simulink model "Test_PMSM_PI_fixed_MTPA"  (R2024b)
settings: Solver=ode45  StartTime=0.0  StopTime=10e-3  FixedStep=Ts  MaxStep=TCs/2  RelTol=1e-3
values from neighbouring files (symbols this model uses):
  Ki_Id = 5.274e3    (= 5274)    [init_params.m]
  Ki_Iq = 9.846e3    (= 9846)    [init_params.m]
  Kp_Id = 4.746    [init_params.m]
  Kp_Iq = 8.861    [init_params.m]
  p = 4    [init_params.m]
  TCs = 1/Fs    (= 0.0001)    [init_params.m]
  Tref = 60    [init_params.m]
undefined symbols (not defined in the file or in its folder): Mot, plecs
libraries: eeTransforms x3, slpidlib x2, simulink x1, spsabctoAlphaBetaZeroLib x1
settings Model: Creator=juan  LastModifiedBy=jd
settings RTWCC: GPUComputeCapability=3.5

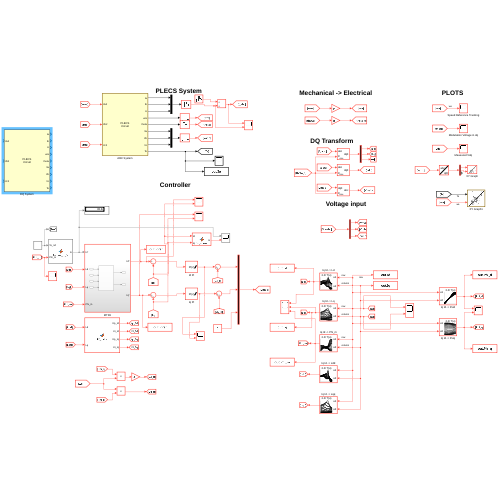
[thumbnail: Simulink's stored preview of the top-level diagram]
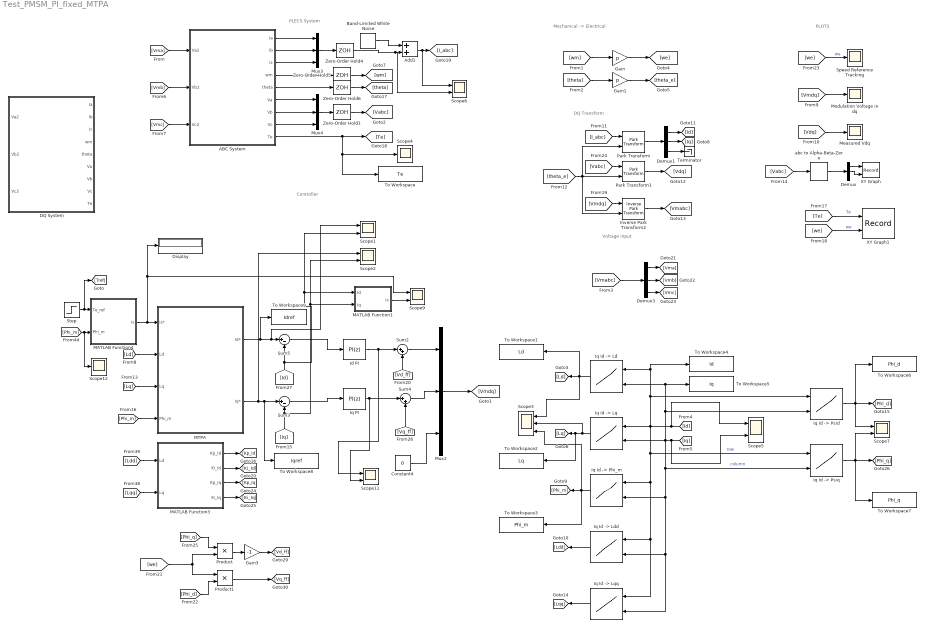
== system Test_PMSM_PI_fixed_MTPA ==
  note: Controller
  note: PLECS System
  note: Mechanical -> Electrical
  note: DQ Transform
  note: PLOTS
  note: Voltage input
  ABC System : Subsystem  LoadFcn=plecs('sl', 200);  InitFcn=plecs('sl', 214);  StartFcn=plecs('sl', 208);  StopFcn=plecs('sl', 209);  mask(PlecsCircuit){PLECSData=<binary blob, 53316 chars, not shown>}
      mask prompts: PLECSData "PLECS Data (Do not delete or modify!)"
      mask init:
      | % PLACE CUSTOM INITIALIZATIONS ABOVE
      | % DO NOT REMOVE
      | plecs('sl', 215);
      | % DO NOT REMOVE
      settings: CopyFcn=plecs('sl', 203);  DeleteFcn=plecs('sl', 205);  UndoDeleteFcn=plecs('sl', 206);  PreSaveFcn=plecs('sl', 211);  PostSaveFcn=plecs('sl', 201);  NameChangeFcn=plecs('sl', 210);  DestroyFcn=plecs('sl', 207);  PreCopyFcn=plecs('sl', 216);  OpenFcn=plecs('sl', 202);  ErrorFcn=plerrorfcn
      mask Help: eval('plecs(''help'', ''qthelp:///creatingacircuit.html'')')
      mask Display: disp('PLECS\nCircuit')
  Add1 : Sum
  Band-Limited White Noise : simulink/Sources/Band-Limited White Noise  Cov=[1]  Ts=TCs  seed=[23341]
  Constant4 : Constant  Value=0  SampleTime=TCs
  DQ System : Subsystem  LoadFcn=plecs('sl', 200);  InitFcn=plecs('sl', 214);  StartFcn=plecs('sl', 208);  StopFcn=plecs('sl', 209);  mask(PlecsCircuit){PLECSData=<binary blob, 50632 chars, not shown>}
      mask prompts: PLECSData "PLECS Data (Do not delete or modify!)"
      mask init:
      | % PLACE CUSTOM INITIALIZATIONS ABOVE
      | % DO NOT REMOVE
      | plecs('sl', 215);
      | % DO NOT REMOVE
      settings: CopyFcn=plecs('sl', 203);  DeleteFcn=plecs('sl', 205);  UndoDeleteFcn=plecs('sl', 206);  PreSaveFcn=plecs('sl', 211);  PostSaveFcn=plecs('sl', 201);  NameChangeFcn=plecs('sl', 210);  DestroyFcn=plecs('sl', 207);  PreCopyFcn=plecs('sl', 216);  OpenFcn=plecs('sl', 202);  ErrorFcn=plerrorfcn
      mask Help: eval('plecs(''help'', ''qthelp:///creatingacircuit.html'')')
      mask Display: disp('PLECS\nCircuit')
  Demux : Demux  Outputs=3
  Demux1 : Demux  Outputs=3
  Demux3 : Demux  Outputs=3
  Display : Display
  Gain : Gain  Gain=p
  Gain1 : Gain  Gain=p
  Gain3 : Gain  Gain=-1
  Id PI : slpidlib/PID Controller  Controller=PI  Form=Parallel  TimeDomain=Discrete-time  UseExternalTs=off  SampleTime=TCs  IntegratorMethod=Forward Euler  FilterMethod=Forward Euler  ControllerParametersSource=internal  P=Kp_Id  I=Ki_Id  UseKiTs=off  D=0  UseExternalDerivativeSource=off  N=100  UseFilter=on  TunerSelectOption=Transfer Function Based (PID Tuner App)  InitialConditionSource=internal  InitialConditionForIntegrator=0  InitialConditionForFilter=0  DifferentiatorICPrevScaledInput=0  ExternalReset=none  TrackingMode=off  Kt=1  LimitOutput=on  SatLimitsSource=internal  UpperSaturationLimit=310/sqrt(3)  LowerSaturationLimit=-310/sqrt(3)  LinearizeAsGain=on  AntiWindupMode=clamping  Kb=1  LimitIntegrator=off  UpperIntegratorSaturationLimit=inf  LowerIntegratorSaturationLimit=-inf  POutMin=[]  POutMax=[]  IOutMin=[]  IOutMax=[]  DOutMin=[]  DOutMax=[]  NOutMin=[]  NOutMax=[]  SumOutMin=[]  SumOutMax=[]  SaturationOutMin=[]  SaturationOutMax=[]  PParamMin=[]  PParamMax=[]  IParamMin=[]  IParamMax=[]  DParamMin=[]  DParamMax=[]  NParamMin=[]  NParamMax=[]  KbParamMin=[]  KbParamMax=[]  KtParamMin=[]  KtParamMax=[]  KbOutMin=[]  KbOutMax=[]  KtOutMin=[]  KtOutMax=[]  IntegratorOutMin=[]  IntegratorOutMax=[]  FilterOutMin=[]  FilterOutMax=[]  SumI1OutMin=[]  SumI1OutMax=[]  SumI2OutMin=[]  SumI2OutMax=[]  SumI3OutMin=[]  SumI3OutMax=[]  SumI4OutMin=[]  SumI4OutMax=[]  SumDOutMin=[]  SumDOutMax=[]  DifferentiatorOutMin=[]  DifferentiatorOutMax=[]  FilterDiffOutCoefMin=[]  FilterDiffOutCoefMax=[]  ReciprocalOutMin=[]  ReciprocalOutMax=[]  SumDenOutMin=[]  SumDenOutMax=[]  SumNumOutMin=[]  SumNumOutMax=[]  DivideOutMin=[]  DivideOutMax=[]  UdiffTsProdOutMin=[]  UdiffTsProdOutMax=[]  NTsProdOutMin=[]  NTsProdOutMax=[]  UintegralTsProdOutMin=[]  UintegralTsProdOutMax=[]  UngainTsProdOutMin=[]  UngainTsProdOutMax=[]  ClampingZeroOutDataTypeStr=Inherit: Inherit via back propagation  ClampingZeroOutMin=[]  ClampingZeroOutMax=[]  FilterDenConstantOutDataTypeStr=Inherit: Inherit via back propagation  FilterDenConstantOutMin=[]  FilterDenConstantOutMax=[]  PCopyOutDataTypeStr=Inherit: Inherit via back propagation  PCopyOutMin=[]  PCopyOutMax=[]  NCopyOutDataTypeStr=Inherit: Inherit via back propagation  NCopyOutMin=[]  NCopyOutMax=[]  IntegratorContinuousStateAttributes=''  IntegratorStateMustResolveToSignalObject=off  IntegratorRTWStateStorageClass=Auto  FilterContinuousStateAttributes=''  FilterStateMustResolveToSignalObject=off  FilterRTWStateStorageClass=Auto  ParallelPVariant=InternalParameters  IdealPVariant=Disabled  IVariant=InternalParameters  DVariant=Disabled  IntegratorVariant=Discrete  SatVariant=Enabled  AWVariant=DiscClampingParallel  PCopyVariant=Disabled  TRVariant=Disabled  FdbkBlocksVariant=Forward  IdealPFdbkVariant=Disabled  SatFdbkVariant=Disabled  DerivativeFilterVariant=Disabled  NVariant=Disabled  NCopyVariant=Disabled_SignalSpec  FilterICVariant=Disabled  IntegratorICVariant=InternalICs  ExternalResetVariant=Disabled  TRSumVariant=Passthrough  SumFdbkVariant=Disabled  SumVariant=Sum_PI  TsampFilterVariant=InternalTs  TsampNgainVariant=Passthrough  TsampIntegralVariant=Disabled_SignalSpec  ExternalSaturationOutDataTypeStr=Inherit: Same as second input  DerivativeSourceVariant=Disabled  PreIntVariant=InternalPreInt
  Inverse Park Transform2 : eeTransforms/Inverse Park Transform  AxisAlignment=D-axis  PowerInvariant=off
      settings: LibrarySourceBlock=|
      | ee_sl_lib/Mathematical
      | Transforms/Inverse
      | Park Transform
  "Iq Id -> Ld" : Lookup_n-D  BreakpointsForDimension1=Mot.mag_t.imd  BreakpointsForDimension2=Mot.mag_t.imq  Table=Mot.mag_t.Lmidd+Mot.mag_t.Lmidq  InternalRulePriority=Speed  RndMeth=Simplest
      settings: InputPortMap=u0,u1
  "Iq Id -> Ldd" : Lookup_n-D  BreakpointsForDimension1=Mot.mag_t.imd  BreakpointsForDimension2=Mot.mag_t.imq  Table=Mot.mag_t.Lmidd  InternalRulePriority=Speed  RndMeth=Simplest
      settings: InputPortMap=u0,u1
  "Iq Id -> Lq" : Lookup_n-D  BreakpointsForDimension1=Mot.mag_t.imd  BreakpointsForDimension2=Mot.mag_t.imq  Table=Mot.mag_t.Lmiqq+Mot.mag_t.Lmidq  InternalRulePriority=Speed  RndMeth=Simplest
      settings: InputPortMap=u0,u1
  "Iq Id -> Lqq" : Lookup_n-D  BreakpointsForDimension1=Mot.mag_t.imd  BreakpointsForDimension2=Mot.mag_t.imq  Table=Mot.mag_t.Lmiqq  InternalRulePriority=Speed  RndMeth=Simplest
      settings: InputPortMap=u0,u1
  "Iq Id -> Phi_m" : Lookup_n-D  BreakpointsForDimension1=Mot.mag_t.imd  BreakpointsForDimension2=Mot.mag_t.imq  Table=Mot.mag_t.Psid - (Mot.mag_t.Lmidd + Mot.mag_t.Lmidq).*Mot.mag_t.imd'  InternalRulePriority=Speed  RndMeth=Simplest
      settings: InputPortMap=u0,u1
  "Iq Id -> Psid" : Lookup_n-D  BreakpointsForDimension1=Mot.mag_t.imd  BreakpointsForDimension2=Mot.mag_t.imq  Table=Mot.mag_t.Psid  InternalRulePriority=Speed  RndMeth=Simplest
      settings: InputPortMap=u0,u1
  "Iq Id -> Psiq" : Lookup_n-D  BreakpointsForDimension1=Mot.mag_t.imd  BreakpointsForDimension2=Mot.mag_t.imq  Table=Mot.mag_t.Psiq  InternalRulePriority=Speed  RndMeth=Simplest
      settings: InputPortMap=u0,u1
  Iq PI : slpidlib/PID Controller  Controller=PI  Form=Parallel  TimeDomain=Discrete-time  UseExternalTs=off  SampleTime=TCs  IntegratorMethod=Forward Euler  FilterMethod=Forward Euler  ControllerParametersSource=internal  P=Kp_Iq  I=Ki_Iq  UseKiTs=off  D=0  UseExternalDerivativeSource=off  N=100  UseFilter=on  TunerSelectOption=Transfer Function Based (PID Tuner App)  InitialConditionSource=internal  InitialConditionForIntegrator=0  InitialConditionForFilter=0  DifferentiatorICPrevScaledInput=0  ExternalReset=none  TrackingMode=off  Kt=1  LimitOutput=on  SatLimitsSource=internal  UpperSaturationLimit=310/sqrt(3)  LowerSaturationLimit=-310/sqrt(3)  LinearizeAsGain=on  AntiWindupMode=clamping  Kb=1  LimitIntegrator=off  UpperIntegratorSaturationLimit=inf  LowerIntegratorSaturationLimit=-inf  POutMin=[]  POutMax=[]  IOutMin=[]  IOutMax=[]  DOutMin=[]  DOutMax=[]  NOutMin=[]  NOutMax=[]  SumOutMin=[]  SumOutMax=[]  SaturationOutMin=[]  SaturationOutMax=[]  PParamMin=[]  PParamMax=[]  IParamMin=[]  IParamMax=[]  DParamMin=[]  DParamMax=[]  NParamMin=[]  NParamMax=[]  KbParamMin=[]  KbParamMax=[]  KtParamMin=[]  KtParamMax=[]  KbOutMin=[]  KbOutMax=[]  KtOutMin=[]  KtOutMax=[]  IntegratorOutMin=[]  IntegratorOutMax=[]  FilterOutMin=[]  FilterOutMax=[]  SumI1OutMin=[]  SumI1OutMax=[]  SumI2OutMin=[]  SumI2OutMax=[]  SumI3OutMin=[]  SumI3OutMax=[]  SumI4OutMin=[]  SumI4OutMax=[]  SumDOutMin=[]  SumDOutMax=[]  DifferentiatorOutMin=[]  DifferentiatorOutMax=[]  FilterDiffOutCoefMin=[]  FilterDiffOutCoefMax=[]  ReciprocalOutMin=[]  ReciprocalOutMax=[]  SumDenOutMin=[]  SumDenOutMax=[]  SumNumOutMin=[]  SumNumOutMax=[]  DivideOutMin=[]  DivideOutMax=[]  UdiffTsProdOutMin=[]  UdiffTsProdOutMax=[]  NTsProdOutMin=[]  NTsProdOutMax=[]  UintegralTsProdOutMin=[]  UintegralTsProdOutMax=[]  UngainTsProdOutMin=[]  UngainTsProdOutMax=[]  ClampingZeroOutDataTypeStr=Inherit: Inherit via back propagation  ClampingZeroOutMin=[]  ClampingZeroOutMax=[]  FilterDenConstantOutDataTypeStr=Inherit: Inherit via back propagation  FilterDenConstantOutMin=[]  FilterDenConstantOutMax=[]  PCopyOutDataTypeStr=Inherit: Inherit via back propagation  PCopyOutMin=[]  PCopyOutMax=[]  NCopyOutDataTypeStr=Inherit: Inherit via back propagation  NCopyOutMin=[]  NCopyOutMax=[]  IntegratorContinuousStateAttributes=''  IntegratorStateMustResolveToSignalObject=off  IntegratorRTWStateStorageClass=Auto  FilterContinuousStateAttributes=''  FilterStateMustResolveToSignalObject=off  FilterRTWStateStorageClass=Auto  ParallelPVariant=InternalParameters  IdealPVariant=Disabled  IVariant=InternalParameters  DVariant=Disabled  IntegratorVariant=Discrete  SatVariant=Enabled  AWVariant=DiscClampingParallel  PCopyVariant=Disabled  TRVariant=Disabled  FdbkBlocksVariant=Forward  IdealPFdbkVariant=Disabled  SatFdbkVariant=Disabled  DerivativeFilterVariant=Disabled  NVariant=Disabled  NCopyVariant=Disabled_SignalSpec  FilterICVariant=Disabled  IntegratorICVariant=InternalICs  ExternalResetVariant=Disabled  TRSumVariant=Passthrough  SumFdbkVariant=Disabled  SumVariant=Sum_PI  TsampFilterVariant=InternalTs  TsampNgainVariant=Passthrough  TsampIntegralVariant=Disabled_SignalSpec  ExternalSaturationOutDataTypeStr=Inherit: Same as second input  DerivativeSourceVariant=Disabled  PreIntVariant=InternalPreInt
  MATLAB Function1 : MATLAB Function  TreatAsAtomicUnit=on
  MATLAB Function3 : MATLAB Function  TreatAsAtomicUnit=on
  MATLAB Function4 : MATLAB Function  TreatAsAtomicUnit=on
  MTPA : Subsystem
  Measured Vdq : Scope
  Modulation Voltage in dq : Scope
  Mux2 : Mux  Inputs=3
  Mux3 : Mux  Inputs=3
  Mux4 : Mux  Inputs=3
  Park Transform : eeTransforms/Park Transform  AxisAlignment=D-axis  PowerInvariant=off
      settings: LibrarySourceBlock=|
      | ee_sl_lib/Mathematical
      | Transforms/Park Transform
  Park Transform1 : eeTransforms/Park Transform  AxisAlignment=D-axis  PowerInvariant=off
      settings: LibrarySourceBlock=|
      | ee_sl_lib/Mathematical
      | Transforms/Park Transform
  Product : Product
  Product1 : Product
  Scope{1..2,5..7,9,11} (7 alike) : Scope  NumInputPorts=2
  Scope12 : Scope
  Scope3 : Scope  NumInputPorts=3
  Scope4 : Scope
  Speed Reference Tracking : Scope
  Step : Step  Time=TCs  After=Tref  SampleTime=0
  Sum2 : Sum  Inputs=|++
  Sum3 : Sum  Inputs=|+-
  Sum4 : Sum  Inputs=|++
  Sum5 : Sum  Inputs=|+-
  Terminator : Terminator
  To Workspace : ToWorkspace  VariableName=Te  SaveFormat=Timeseries  SampleTime=-1
  To Workspace1 : ToWorkspace  VariableName=Ld  SaveFormat=Timeseries  SampleTime=-1
  To Workspace2 : ToWorkspace  VariableName=Lq  SaveFormat=Timeseries  SampleTime=-1
  To Workspace3 : ToWorkspace  VariableName=Phi_m  SaveFormat=Timeseries  SampleTime=-1
  To Workspace4 : ToWorkspace  VariableName=Id  SaveFormat=Timeseries  SampleTime=-1
  To Workspace5 : ToWorkspace  VariableName=Iq  SaveFormat=Timeseries  SampleTime=-1
  To Workspace6 : ToWorkspace  VariableName=Phi_d  SaveFormat=Timeseries  SampleTime=-1
  To Workspace7 : ToWorkspace  VariableName=Phi_q  SaveFormat=Timeseries  SampleTime=-1
  To Workspace8 : ToWorkspace  VariableName=Iqref  SaveFormat=Timeseries  SampleTime=-1
  To Workspace9 : ToWorkspace  VariableName=Idref  SaveFormat=Timeseries  SampleTime=-1
  XY Graph : Record  FileSettingsInternal="{\"entries\":[{\"content\":{\"excelSettings\":{\"content\":{},\"type\":\"Streamout.ExcelSettings\"}},\"type\":\"Streamout.FileSettingStorage\",\"uuid\":\"\"}],\"packageUris\":[\"http:\\/\\/schema.mathworks.com\\/mf0\\/streamout_blocks\\/R2020a\"],\"version\":\"1.0\"}"  Layout=[1 1]  SignalsInternal="{\"entries\":[{\"content\":{\"signals\":[{\"content\":{\"blockPath\":[],\"dimensions\":[1],\"domain\":\"\",\"lineColor\":\"#a2142f\",\"plots\":[ 1 ],\"port\":1,\"sid\":[\"\"],\"signalID\":1,\"signalName\":\"Demux:1\"},\"type\":\"RecordBlkView.Signal\",\"uuid\":\"\"},{\"content\":{\"blockPath\":[],\"dimensions\":[1],\"domain\":\"\",\"lineColor\":\"#139fff\",\"plots\":[ 1 ],\"port\":2,\"sid\":[\"\"],\"signalID\":2,\"signalName\":\"Demux:2\"},\"type\":\"RecordBlkView.Signal\",\"uuid\":\"\"}]},\"type\":\"RecordBlkView.InputSignals\",\"uuid\":\"\"}],\"packageUris\":[\"http:\\/\\/schema.mathworks.com\\/mf0\\/streamout_blocks\\/R2020a\"],\"version\":\"1.0\"}"  VisualizationBindings="{\"xyplotplugin\":{\"info\":[{\"series\":[{\"bindingParametersList\":[{\"parameter\":\"X-Axis\",\"signalID\":1,\"signalName\":\"Demux:1\"},{\"parameter\":\"Y-Axis\",\"signalID\":2,\"signalName\":\"Demux:2\"}],\"seriesID\":0}],\"subplotID\":1}]}}"  CompatibilityTag=XY
  XY Graph1 : Record  FileSettingsInternal="{\"entries\":[{\"content\":{\"excelSettings\":{\"content\":{},\"type\":\"Streamout.ExcelSettings\"}},\"type\":\"Streamout.FileSettingStorage\",\"uuid\":\"\"}],\"packageUris\":[\"http:\\/\\/schema.mathworks.com\\/mf0\\/streamout_blocks\\/R2020a\"],\"version\":\"1.0\"}"  Layout=[1 1]  SignalsInternal="{\"entries\":[{\"content\":{\"signals\":[{\"content\":{\"blockPath\":[],\"dimensions\":[1],\"domain\":\"\",\"lineColor\":\"#a2142f\",\"plots\":[ 1 ],\"port\":1,\"sid\":[\"\"],\"signalID\":1,\"signalName\":\"Te\"},\"type\":\"RecordBlkView.Signal\",\"uuid\":\"\"},{\"content\":{\"blockPath\":[],\"dimensions\":[1],\"domain\":\"\",\"lineColor\":\"#139fff\",\"plots\":[ 1 ],\"port\":2,\"sid\":[\"\"],\"signalID\":2,\"signalName\":\"we\"},\"type\":\"RecordBlkView.Signal\",\"uuid\":\"\"}]},\"type\":\"RecordBlkView.InputSignals\",\"uuid\":\"\"}],\"packageUris\":[\"http:\\/\\/schema.mathworks.com\\/mf0\\/streamout_blocks\\/R2020a\"],\"version\":\"1.0\"}"  VisualizationBindings="{\"xyplotplugin\":{\"info\":[{\"series\":[{\"bindingParametersList\":[{\"parameter\":\"X-Axis\",\"signalID\":2,\"signalName\":\"we\"},{\"parameter\":\"Y-Axis\",\"signalID\":1,\"signalName\":\"Te\"}],\"seriesID\":0}],\"subplotID\":1}]}}"  CompatibilityTag=XY
  Zero-Order Hold{1,4..6} (4 alike) : ZeroOrderHold  SampleTime=TCs
  abc to Alpha-Beta-Zero : spsabctoAlphaBetaZeroLib/abc to Alpha-Beta-Zero
  wires:
  [Vma] -> ABC System/1(Va2)
  [wm] -> Gain/1
  Gain/1 -> [we]
  [theta] -> Gain1/1
  Gain1/1 -> [theta_e]
  [Vmb] -> ABC System/2(Vb2)
  [Vmc] -> ABC System/3(Vc2)
  [I_abc] -> Park Transform/1
  Park Transform/1 -> Demux1/1
  Demux1/1 -> [Id]
  Demux1/2 -> [Iq]
  Demux1/3 -> Terminator/1
  [Vmdq] -> Inverse Park Transform2/1
  Inverse Park Transform2/1 -> [Vmabc]
  [we] -> Speed Reference Tracking/1  "we"
  [Vabc] -> Park Transform1/1
  [theta_e] -> Inverse Park Transform2/2, Park Transform1/2, Park Transform/2
  Park Transform1/1 -> [Vdq]
  [Vmdq] -> Modulation Voltage in dq/1
  [Vdq] -> Measured Vdq/1
  [Vabc] -> abc to Alpha-Beta-Zero/1
  abc to Alpha-Beta-Zero/1 -> Demux/1
  Demux/1 -> XY Graph/1
  Demux/2 -> XY Graph/2
  ABC System/4(wm) -> Zero-Order Hold5/1
  Mux3/1 -> Zero-Order Hold4/1
  Mux4/1 -> Zero-Order Hold1/1
  ABC System/6(Va) -> Mux4/1
  ABC System/7(Vb) -> Mux4/2
  ABC System/9(Te) -> To Workspace/1, Scope4/1, [Te]
  ABC System/3(Ic) -> Mux3/3
  Zero-Order Hold5/1 -> [wm]
  Zero-Order Hold6/1 -> [theta]
  ABC System/5(theta) -> Zero-Order Hold6/1
  ABC System/8(Vc) -> Mux4/3
  ABC System/2(Ib) -> Mux3/2
  ABC System/1(Ia) -> Mux3/1
  [Id] -> Scope5/1, "Iq Id -> Lqq"/1, "Iq Id -> Ldd"/1, "Iq Id -> Phi_m"/1, "Iq Id -> Psiq"/1, "Iq Id -> Psid"/1, "Iq Id -> Ld"/1, To Workspace4/1, "Iq Id -> Lq"/1  "row"
  [Iq] -> Scope5/2, "Iq Id -> Psiq"/2, "Iq Id -> Lqq"/2, "Iq Id -> Ldd"/2, "Iq Id -> Phi_m"/2, "Iq Id -> Psid"/2, "Iq Id -> Ld"/2, To Workspace5/1, "Iq Id -> Lq"/2  "column"
  "Iq Id -> Ld"/1 -> To Workspace1/1, Scope3/1, [Ld]
  [Ld] -> MTPA/2(Ld)
  [Lq] -> MTPA/3(Lq)
  Step/1 -> MATLAB Function4/1(Te_ref), [Tref]
  "Iq Id -> Phi_m"/1 -> To Workspace3/1, Scope3/3, [Phi_m]
  [Phi_m] -> MTPA/4(Phi_m)
  "Iq Id -> Lq"/1 -> To Workspace2/1, [Lq], Scope3/2
  [Te] -> XY Graph1/1  "Te"
  [we] -> XY Graph1/2  "we"
  "Iq Id -> Psid"/1 -> Scope7/1, To Workspace6/1, [Phi_d]
  "Iq Id -> Psiq"/1 -> To Workspace7/1, [Phi_q], Scope7/2
  Zero-Order Hold1/1 -> [Vabc]
  Demux3/2 -> [Vmb]
  Demux3/3 -> [Vmc]
  [Vmabc] -> Demux3/1
  Demux3/1 -> [Vma]
  [Lqq] -> MATLAB Function3/2(Lq)
  [Ldd] -> MATLAB Function3/1(Ld)
  MATLAB Function1/1(Is) -> Scope9/2
  Sum5/1 -> Id PI/1
  [Iq] -> Scope2/2, MATLAB Function1/2(Iq), Sum3/2
  MATLAB Function3/1(Kp_Id) -> [Kp_Id]
  MATLAB Function3/2(Ki_Id) -> [Ki_Id]
  MATLAB Function3/3(Kp_Iq) -> [Kp_Iq]
  MATLAB Function3/4(Ki_Iq) -> [Ki_Iq]
  MTPA/1(Id*) -> To Workspace9/1, Scope1/1, Sum5/1
  MTPA/2(Iq*) -> To Workspace8/1, Sum3/1, Scope2/1
  Sum3/1 -> Iq PI/1
  "Iq Id -> Ldd"/1 -> [Ldd]
  "Iq Id -> Lqq"/1 -> [Lqq]
  [Id] -> Scope1/2, MATLAB Function1/1(Id), Sum5/2
  MATLAB Function4/1(Is) -> Display/1, Scope9/1, MTPA/1(Is*)
  [Phi_m] -> Scope12/1, MATLAB Function4/2(Phi_m)
  Gain3/1 -> [Vd_ff]
  [Phi_q] -> Product/1
  Product1/1 -> [Vq_ff]
  [we] -> Product1/1, Product/2
  [Phi_d] -> Product1/2
  Product/1 -> Gain3/1
  Iq PI/1 -> Scope11/2, Sum4/1
  Constant4/1 -> Mux2/3
  Mux2/1 -> [Vmdq]
  Sum4/1 -> Mux2/2
  [Vd_ff] -> Sum2/2
  Sum2/1 -> Mux2/1
  Id PI/1 -> Sum2/1, Scope11/1
  [Vq_ff] -> Sum4/2
  Add1/1 -> Scope6/1, [I_abc]
  Band-Limited White Noise/1 -> Add1/1
  Zero-Order Hold4/1 -> Scope6/2, Add1/2

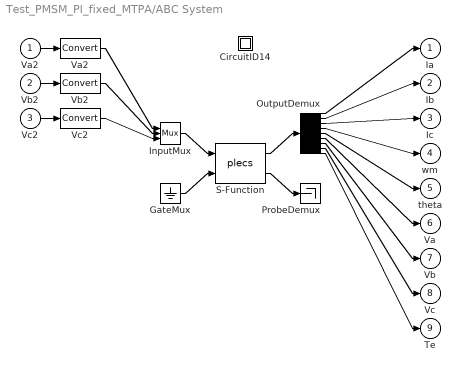
== system Test_PMSM_PI_fixed_MTPA/ABC System ==
  Va2 : Inport  PortDimensions=1
  Vb2 : Inport  Port=2  PortDimensions=1
  Vc2 : Inport  Port=3  PortDimensions=1
  " CircuitID14 " : Subsystem
  " GateMux " : Ground
  " InputMux " : Mux  Inputs=[ 1 1 1 ]
  " OutputDemux " : Demux  Outputs=[ 1 1 1 1 1 1 1 1 1 ]
  " ProbeDemux " : Terminator
  " S-Function " : S-Function  FunctionName=plecs  SFunctionDeploymentMode=off  EnableBusSupport=off
  " Va2 " : DataTypeConversion
  " Vb2 " : DataTypeConversion
  " Vc2 " : DataTypeConversion
  Ia : Outport  PortDimensions=1
  Ib : Outport  Port=2  PortDimensions=1
  Ic : Outport  Port=3  PortDimensions=1
  wm : Outport  Port=4  PortDimensions=1
  theta : Outport  Port=5  PortDimensions=1
  Va : Outport  Port=6  PortDimensions=1
  Vb : Outport  Port=7  PortDimensions=1
  Vc : Outport  Port=8  PortDimensions=1
  Te : Outport  Port=9  PortDimensions=1
  wires:
  " InputMux "/1 -> " S-Function "/1
  " GateMux "/1 -> " S-Function "/2
  " S-Function "/1 -> " OutputDemux "/1
  " S-Function "/2 -> " ProbeDemux "/1
  Va2/1 -> " Va2 "/1
  " Va2 "/1 -> " InputMux "/1
  Vb2/1 -> " Vb2 "/1
  " Vb2 "/1 -> " InputMux "/2
  Vc2/1 -> " Vc2 "/1
  " Vc2 "/1 -> " InputMux "/3
  " OutputDemux "/1 -> Ia/1
  " OutputDemux "/2 -> Ib/1
  " OutputDemux "/3 -> Ic/1
  " OutputDemux "/4 -> wm/1
  " OutputDemux "/5 -> theta/1
  " OutputDemux "/6 -> Va/1
  " OutputDemux "/7 -> Vb/1
  " OutputDemux "/8 -> Vc/1
  " OutputDemux "/9 -> Te/1

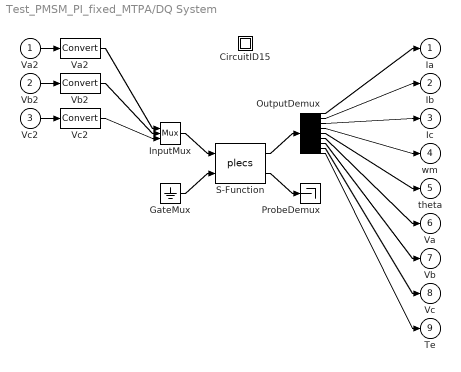
== system Test_PMSM_PI_fixed_MTPA/DQ System ==
  Va2 : Inport  PortDimensions=1
  Vb2 : Inport  Port=2  PortDimensions=1
  Vc2 : Inport  Port=3  PortDimensions=1
  " CircuitID15 " : Subsystem
  " GateMux " : Ground
  " InputMux " : Mux  Inputs=[ 1 1 1 ]
  " OutputDemux " : Demux  Outputs=[ 1 1 1 1 1 1 1 1 1 ]
  " ProbeDemux " : Terminator
  " S-Function " : S-Function  FunctionName=plecs  SFunctionDeploymentMode=off  EnableBusSupport=off
  " Va2 " : DataTypeConversion
  " Vb2 " : DataTypeConversion
  " Vc2 " : DataTypeConversion
  Ia : Outport  PortDimensions=1
  Ib : Outport  Port=2  PortDimensions=1
  Ic : Outport  Port=3  PortDimensions=1
  wm : Outport  Port=4  PortDimensions=1
  theta : Outport  Port=5  PortDimensions=1
  Va : Outport  Port=6  PortDimensions=1
  Vb : Outport  Port=7  PortDimensions=1
  Vc : Outport  Port=8  PortDimensions=1
  Te : Outport  Port=9  PortDimensions=1
  wires:
  " InputMux "/1 -> " S-Function "/1
  " GateMux "/1 -> " S-Function "/2
  " S-Function "/1 -> " OutputDemux "/1
  " S-Function "/2 -> " ProbeDemux "/1
  Va2/1 -> " Va2 "/1
  " Va2 "/1 -> " InputMux "/1
  Vb2/1 -> " Vb2 "/1
  " Vb2 "/1 -> " InputMux "/2
  Vc2/1 -> " Vc2 "/1
  " Vc2 "/1 -> " InputMux "/3
  " OutputDemux "/1 -> Ia/1
  " OutputDemux "/2 -> Ib/1
  " OutputDemux "/3 -> Ic/1
  " OutputDemux "/4 -> wm/1
  " OutputDemux "/5 -> theta/1
  " OutputDemux "/6 -> Va/1
  " OutputDemux "/7 -> Vb/1
  " OutputDemux "/8 -> Vc/1
  " OutputDemux "/9 -> Te/1

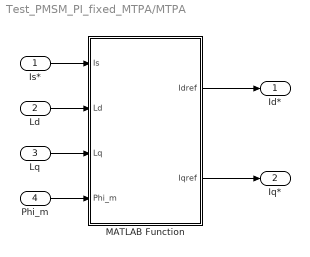
== system Test_PMSM_PI_fixed_MTPA/MTPA ==
  Is* : Inport
  Ld : Inport  Port=2
  Lq : Inport  Port=3
  Phi_m : Inport  Port=4
  MATLAB Function : MATLAB Function  TreatAsAtomicUnit=on
  Id* : Outport
  Iq* : Outport  Port=2
  wires:
  Lq/1 -> MATLAB Function/3(Lq)
  Ld/1 -> MATLAB Function/2(Ld)
  MATLAB Function/1(Idref) -> Id*/1
  MATLAB Function/2(Iqref) -> Iq*/1
  Is*/1 -> MATLAB Function/1(Is)
  Phi_m/1 -> MATLAB Function/4(Phi_m)

== system Test_PMSM_PI_fixed_MTPA/ABC System/ CircuitID14  ==

== system Test_PMSM_PI_fixed_MTPA/DQ System/ CircuitID15  ==

== matlab function Test_PMSM_PI_fixed_MTPA/MTPA/MATLAB Function ==
  settings: updateMethod=DISCRETE  sampleTime=TCs
  data: Is input; Ld input; Lq input; Phi_m input; Idref output; Iqref output
function [Idref, Iqref] = MTPA(Is, Ld, Lq, Phi_m)

if Lq > Ld
    Idref = (Phi_m - sqrt(Phi_m^2 + 8*(Lq - Ld)^2*Is^2))/(4*(Lq - Ld));
    Idref = min(max(Idref, -Is), 0);
    Iqref = sign(Is)*sqrt(Is^2 - Idref^2);
else
    Idref = 0;
    Iqref = Is;
end

== matlab function Test_PMSM_PI_fixed_MTPA/MATLAB Function1 ==
  data: Id input; Is output; Iq input
function Is = Is_norm(Id, Iq)
Is = sqrt(Id^2 + Iq^2);

== matlab function Test_PMSM_PI_fixed_MTPA/MATLAB Function3 ==
  settings: updateMethod=DISCRETE  sampleTime=TCs
  data: Ld input; Kp_Id output; Lq input; Ki_Id output; Kp_Iq output; Ki_Iq output; TCs parameter
function [Kp_Id, Ki_Id, Kp_Iq, Ki_Iq] = PI_gains(Ld, Lq, TCs)
    k = 3; % 3 based on paper

    % Ts = TCs; L = Ldq; 
    % Kp = L/(k*Ts) -- Ki = L/(k^3*Ts^2)
    Kp_Id = Ld/(k*TCs);
    Ki_Id = Ld/(k^3*TCs^2);
    Kp_Iq = Lq/(k*TCs);
    Ki_Iq = Lq/(k^3*TCs^2);
end

== matlab function Test_PMSM_PI_fixed_MTPA/MATLAB Function4 ==
  data: Te_ref input; Is output; Phi_m input; p parameter
function Is = Torque_to_Is(Te_ref, Phi_m, p)
% PLECS data - 60 Nm
% Is = 0.9*Te_ref*2/(3*p*Phi_m);
if Te_ref == 60
    % Hande FEM data - 60 Nm
    Is = 0.877*Te_ref*2/(3*p*Phi_m);
elseif Te_ref == 120
    % Hande FEM data - 120 Nm
    Is = 1.007*Te_ref*2/(3*p*Phi_m);
else
    Is = 1*Te_ref*2/(3*p*Phi_m);
% Hande Greybox data - 60 Nm
% Is = 1.25*Te_ref*2/(3*p*Phi_m);
end
